simulink model "ARCH_AT2"  (R2019b)
settings: Solver=FixedStepAuto  StartTime=0.0  StopTime=10.0  FixedStep=fixedStepSize  RelTol=1e-3
undefined symbols (not defined in the file): ARCH_AT2_rpmLimit, ARCH_AT2_rpmLimitAct
settings Model: Creator=JEDDELAN  LastModifiedBy=alex
settings DataIOCC: SaveOutput=off  SaveTime=off  ReturnWorkspaceOutputs=off
settings DebuggingCC: ArithmeticOperatorsInVariantConditions=warning
settings SFSimCC: SimUseLocalCustomCode=off  CustomCodeUndefinedFunction=UseInterfaceOnly
settings RTWCC: RTWUseLocalCustomCode=off
settings GRTTargetCC: CombineOutputUpdateFcns=off  MatFileLogging=off

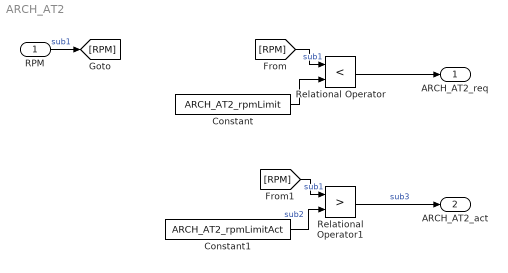
== system ARCH_AT2 ==
  RPM : Inport
  Constant : Constant  Value=ARCH_AT2_rpmLimit
  Constant1 : Constant  Value=ARCH_AT2_rpmLimitAct
  Relational Operator : RelationalOperator  Operator=<  OutDataTypeStr=boolean  RndMeth=Simplest
  Relational Operator1 : RelationalOperator  Operator=>  OutDataTypeStr=boolean  RndMeth=Simplest
  ARCH_AT2_req : Outport  OutDataTypeStr=boolean  PortDimensions=1  VectorParamsAs1DForOutWhenUnconnected=off
  ARCH_AT2_act : Outport  Port=2  OutDataTypeStr=boolean  PortDimensions=1  VectorParamsAs1DForOutWhenUnconnected=off
  wires:
  RPM/1 -> [RPM]  "sub1"
  Constant/1 -> Relational Operator/2
  [RPM] -> Relational Operator/1  "sub1"
  Relational Operator/1 -> ARCH_AT2_req/1
  Constant1/1 -> Relational Operator1/2  "sub2"
  [RPM] -> Relational Operator1/1  "sub1"
  Relational Operator1/1 -> ARCH_AT2_act/1  "sub3"
